simulink model "Simulacion_stepper"  (R2025b)
settings: Solver=ode4  StartTime=0.0  StopTime=Time_simulation  FixedStep=1/frecuency_simulation  RelTol=1e-3
InitFcn:
  | %%InitFcn();
StopFcn:
  | %%FinishFcn
model workspace (MAT data in the model file):
  Ts_stepper = 0.001
values from neighbouring files (symbols this model uses):
  B = motor_params.B_internal    [bode.m]    (also in current_observer.m = 0.0005; discretizacion.m = [ 1/L, 0; ekf_4_estados.m = params.B; obs_ctrl_back_emf_ext.m = [1/L 0)
  frecuency_simulation = 10e3    (= 10000)    [InitFcn.m]
  J = motor_params.J_internal    [bode.m]    (also in current_observer.m = 0.008; ekf_4_estados.m = params.J; obs_ctrl_back_emf_ext.m = 0.008; obs_y_contrl_back_emd.m = 0.008)
  Ke = 0.0055    [current_observer.m]    (also in ekf_4_estados.m = params.Ke; observer.m = Pvec(3); salient_motor.m = 0.0066)
  Ki_d = PI_dq_params.Ki_d_salient    [bode.m]
  Ki_q = PI_dq_params.Ki_q_salient    [bode.m]
  Ki_w = (wn_w^2)*J_var/Kt    [Barrido_B.m]    (also in Barrido_J.m; bode.m = PI_MTPA_params.Ki_w)
  Kp_d = PI_dq_params.Kp_d_salient    [bode.m]
  Kp_q = PI_dq_params.Kp_q_salient    [bode.m]
  Kp_w = (2*shi_w*wn_w*J_var)/Kt    [Barrido_B.m]    (also in Barrido_J.m; bode.m = PI_MTPA_params.Kp_w)
  Kt = Nr*Ke    (= 0.275)    [current_observer.m]    (also in ekf_4_estados.m = params.Kt; frecuencia_max.m = 0.33; observer.m = Pvec(4); salient_motor.m = 0.33)
  L = place(A', C', 10*eig(A)).'    [current_observer.m]    (also in desfase.m = lags(k); discretizacion.m = 0.01; frecuencia_max.m = 0.006; obs_ctrl_back_emf_ext.m = 0.006)
  P = motor_params.P    [bode.m]    (also in ekf_4_estados.m = P_pred; frecuencia_max.m = 50; salient_motor.m = 50)
  R = motor_params.R    [bode.m]    (also in current_observer.m = 3.4; discretizacion.m = 3.4; ekf_4_estados.m = params.R; frecuencia_max.m = 3.4)
  sample_time = 1/frecuency_simulation    (= 0.0001)    [InitFcn.m]
  Ts_current = 1/f_current    (= 0.0001)    [InitFcn.m]
  Ts_Wm = Ts_current*10    (= 0.001)    [InitFcn.m]
  Vdc = 24    [InitFcn.m]    (also in frecuencia_max.m = 12)
undefined symbols (not defined in the file or in its folder): DiscIntNeverNeededParam, EKF_params, motor_params, RI_base
libraries: simulink x8, mcbeeMathTransformLib x3, spspowerguiLib x1
(part 5 of 5)

== matlab function Simulacion_stepper/Triggered Subsystem1/MATLAB Function ==
  data: U input; x_out output; X input; Ts input; Ke input; Kt input; R input; J input; Ld input; Lq input; Nr input; B input; wh input; b0 input; b1 input; b2 input; a1 input; a2 input; HFI_flag input
function x_out = ekf_dq_5states_tightly_coupled( ...
    U, X, Ts, Ke, Kt, R, J, Ld, Lq, Nr, B, ...
    wh, b0, b1, b2, a1, a2, HFI_flag)

% =========================================================================
% EKF 5 ESTADOS TIGHTLY COUPLED CON HFI
%
% Estados:
%
%   x = [Id; Iq; Wm; theta_e; Tx]
%
% theta_e:
%   Ángulo eléctrico.
%
% Mediciones:
%
%   y_med  = [Ia; Ib; 0]
%   y_pred = [Ia_pred; Ib_pred; eps_norm]
%
% La tercera medición impone:
%
%   eps_norm -> 0
%
% IMPORTANTE:
%   Para que esta formulación sea físicamente coherente, eps_norm debe
%   representar aproximadamente un error angular eléctrico.
% =========================================================================

% Parámetros no utilizados actualmente:
% N_steps, Tdtm, beta0, beta1, beta2

Ts_eff = max(Ts, 1e-9);

% =========================================================================
% ESTADOS PERSISTENTES
% =========================================================================

persistent x_hat
persistent P
persistent Qk

persistent xa1 xa2 ya1 ya2
persistent xb1 xb2 yb1 yb2

persistent t_h
persistent eps_f

if isempty(x_hat)

    % Estado inicial
    x_hat = zeros(5,1);

    % Covarianza inicial
    P = diag([ ...
        1e-6, ...   % Id
        1e-6, ...   % Iq
        1e-6, ...   % Wm
        1e-9, ...   % theta_e
        1e-5]);     % Tx

    % Ruido del proceso
    Qk = diag([ ...
        1e-8, ...   % Id
        1e-8, ...   % Iq
        1e-8, ...   % Wm
        1e-12, ...   % theta_e
        1e-5]);     % Tx

    % Estados del BPF de Ia
    xa1 = 0;
    xa2 = 0;
    ya1 = 0;
    ya2 = 0;

    % Estados del BPF de Ib
    xb1 = 0;
    xb2 = 0;
    yb1 = 0;
    yb2 = 0;

    % Estados HFI
    t_h   = 0;
    eps_f = 0;

end

% =========================================================================
% 1. MEDICIONES Y ENTRADAS
% =========================================================================

Ia_raw = X(1);
Ib_raw = X(2);

Va = U(1);
Vb = U(2);

% =========================================================================
% 2. ESTADOS ACTUALES
% =========================================================================

Id = x_hat(1);
Iq = x_hat(2);
Wm = x_hat(3);

% El estado angular se conserva continuo internamente
theta_e_state = x_hat(4);

Tx = x_hat(5);

% Ángulo envuelto únicamente para trigonometría
theta_e = wrap_pi(theta_e_state);

c = cos(theta_e);
s = sin(theta_e);

% =========================================================================
% 3. TRANSFORMACIÓN DE TENSIONES AL MARCO dq
% =========================================================================

Vd =  Va*c + Vb*s;
Vq = -Va*s + Vb*c;

% =========================================================================
% 4. PREDICCIÓN DEL ESTADO
% =========================================================================

We = Nr*Wm;

dId = ( ...
      Vd ...
    - R*Id ...
    + We*Lq*Iq) / Ld;

dIq = ( ...
      Vq ...
    - R*Iq ...
    - We*Ld*Id ...
    - Ke*Wm) / Lq;

% Torque electromagnético
Te = Kt*Iq + Nr*(Lq-Ld)*Id*Iq;

% Tx representa la carga desconocida
dWm = (Te - B*Wm - Tx)/J;

% Alternativa si Tdtm es una carga conocida:
%
% dWm = (Te - B*Wm - Tdtm - Tx)/J;

x_pred = zeros(5,1);

x_pred(1) = Id + Ts_eff*dId;
x_pred(2) = Iq + Ts_eff*dIq;
x_pred(3) = Wm + Ts_eff*dWm;

% Ángulo eléctrico continuo
x_pred(4) = theta_e_state + Ts_eff*Nr*Wm;

% Torque desconocido como random walk
x_pred(5) = Tx;

% =========================================================================
% 5. JACOBIANA DE TRANSICIÓN
% =========================================================================

A = [ ...
    -R/Ld, ...
     Nr*Wm*Lq/Ld, ...
     Nr*Lq*Iq/Ld, ...
     Vq/Ld, ...
     0;

    -Nr*Wm*Ld/Lq, ...
    -R/Lq, ...
    -(Nr*Ld*Id + Ke)/Lq, ...
    -Vd/Lq, ...
     0;

     Nr*(Lq-Ld)*Iq/J, ...
     (Kt + Nr*(Lq-Ld)*Id)/J, ...
    -B/J, ...
     0, ...
    -1/J;

     0, ...
     0, ...
     Nr, ...
     0, ...
     0;

     0, ...
     0, ...
     0, ...
     0, ...
     0];

Phi = eye(5) + Ts_eff*A;

P_pred = Phi*P*Phi' + Qk;
P_pred = 0.5*(P_pred + P_pred');

% =========================================================================
% 6. FILTRO PASABANDA DE LAS CORRIENTES HFI
% =========================================================================

Iah = ...
      b0*Ia_raw ...
    + b1*xa1 ...
    + b2*xa2 ...
    - a1*ya1 ...
    - a2*ya2;

xa2 = xa1;
xa1 = Ia_raw;

ya2 = ya1;
ya1 = Iah;

Ibh = ...
      b0*Ib_raw ...
    + b1*xb1 ...
    + b2*xb2 ...
    - a1*yb1 ...
    - a2*yb2;

xb2 = xb1;
xb1 = Ib_raw;

yb2 = yb1;
yb1 = Ibh;

% =========================================================================
% 7. PROYECCIÓN HFI RESPECTO DEL ÁNGULO PREDICHO
% =========================================================================

theta_e_pred = wrap_pi(x_pred(4));

ch = cos(theta_e_pred);
sh = sin(theta_e_pred);

% Componente HFI sobre el eje q estimado
Iqh = -Iah*sh + Ibh*ch;

% =========================================================================
% 8. DEMODULACIÓN SÍNCRONA
% =========================================================================

if wh > 0

    t_h = t_h + Ts_eff;

    T_hfi = 2*pi/wh;

    if t_h >= T_hfi
        t_h = t_h - T_hfi*floor(t_h/T_hfi);
    end

    % Verificar signo y fase según la señal efectivamente inyectada
    eps_raw = -Iqh*cos(wh*t_h);

else

    t_h = 0;
    eps_raw = 0;

end

% =========================================================================
% 9. FILTRO PASABAJOS DEL ERROR HFI
% =========================================================================

f_lpf_hfi = 50;

tau_lpf   = 1/(2*pi*f_lpf_hfi);
alpha_lpf = Ts_eff/(Ts_eff + tau_lpf);

eps_f = eps_f + alpha_lpf*(eps_raw - eps_f);

% =========================================================================
% 10. NORMALIZACIÓN DEL ERROR HFI
% =========================================================================

DeltaL = Lq - Ld;
Lavg   = 0.5*(Ld + Lq);

if abs(DeltaL) < 1e-12 || Lavg <= 0

    eps_norm = 0;

else

    saliency = DeltaL/Lavg;

    % Formulación original:
    %
    % Se supone empíricamente que eps_norm aproxima un error angular.
    %
    % Atención: dividir por la saliencia no garantiza que el resultado
    % tenga unidades de radianes.
    % Formulación original:
    eps_norm = eps_f/abs(saliency);
    
    % NUEVO: Límite estricto de seguridad para evitar retroalimentación positiva
    max_eps = pi/4; % 45 grados eléctricos
    eps_norm = max(-max_eps, min(max_eps, eps_norm));

end

if ~HFI_flag
    eps_norm = 0;
end

% Protección numérica
if ~isfinite(eps_norm)
    eps_norm = 0;
end

% =========================================================================
% 11. PREDICCIÓN DE LAS MEDICIONES DE CORRIENTE
% =========================================================================

Id_p = x_pred(1);
Iq_p = x_pred(2);

cp = cos(theta_e_pred);
sp = sin(theta_e_pred);

Ia_pred = Id_p*cp - Iq_p*sp;
Ib_pred = Id_p*sp + Iq_p*cp;

% =========================================================================
% 12. VECTOR DE MEDICIÓN DE TRES COMPONENTES
% =========================================================================
%
% La tercera medición impone que el error HFI sea cero.
% =========================================================================

y_med = [ ...
    Ia_raw;
    Ib_raw;
    0];

y_pred = [ ...
    Ia_pred;
    Ib_pred;
    eps_norm];

innov = y_med - y_pred;

% Equivalente:
%
% innov(1) = Ia_raw - Ia_pred
% innov(2) = Ib_raw - Ib_pred
% innov(3) = -eps_norm

% =========================================================================
% 13. JACOBIANA DE MEDICIÓN
% =========================================================================

dIa_dtheta_e = -Id_p*sp - Iq_p*cp;
dIb_dtheta_e =  Id_p*cp - Iq_p*sp;

% Si:
%
% eps_norm ≈ theta_real - theta_estimado
%
% entonces:
%
% d(eps_norm)/d(theta_estimado) ≈ -1
dEps_dtheta_e = -1;

Ck = [ ...
    cp, -sp, 0, dIa_dtheta_e, 0;
    sp,  cp, 0, dIb_dtheta_e, 0;
    0,   0,  0, dEps_dtheta_e, 0];

% =========================================================================
% 14. COVARIANZA DE LAS TRES MEDICIONES
% =========================================================================

sigma_Ia = 0.1;
sigma_Ib = 0.1;

if HFI_flag

    sigma_HFI = 0.25;

else

    % El HFI queda prácticamente ignorado
    sigma_HFI = 1e6;

end

Rk = diag([ ...
    sigma_Ia^2, ...
    sigma_Ib^2, ...
    sigma_HFI^2]);

% =========================================================================
% 15. GANANCIA DE KALMAN
% =========================================================================

Sk = Ck*P_pred*Ck' + Rk;
Sk = 0.5*(Sk + Sk');

% Evitar inversión explícita
Lk = (P_pred*Ck')/Sk;

% =========================================================================
% 16. CORRECCIÓN TIGHTLY COUPLED
% =========================================================================

x_corr_ekf = x_pred + Lk*innov;

% No se envuelve internamente para mantener continuidad angular
% x_corr_ekf(4) permanece continuo.

% =========================================================================
% 17. ACTUALIZACIÓN DE COVARIANZA: FORMA DE JOSEPH
% =========================================================================

I5 = eye(5);

P = ...
    (I5 - Lk*Ck)*P_pred*(I5 - Lk*Ck)' ...
    + Lk*Rk*Lk';

P = 0.5*(P + P');

% =========================================================================
% 18. PROTECCIÓN NUMÉRICA
% =========================================================================

if any(~isfinite(x_corr_ekf)) || any(~isfinite(P(:)))

    x_corr_ekf = x_pred;
    P = P_pred;

end

% =========================================================================
% 19. ACTUALIZACIÓN DEL ESTADO
% =========================================================================

x_hat = x_corr_ekf;

% =========================================================================
% 20. SALIDA
% =========================================================================

x_out = x_hat;

% Solo la salida angular se envuelve
x_out(4) = wrap_pi(x_hat(4));

end

% =========================================================================
% FUNCIÓN AUXILIAR
% =========================================================================

function out = wrap_pi(in)

out = atan2(sin(in), cos(in));

end
